simulink model "PIcontroller"  (R2014b)
settings: Solver=ode15s  StartTime=0.0  StopTime=10.0  RelTol=1e-3
settings Model: Creator=c412  LastModifiedBy=c412

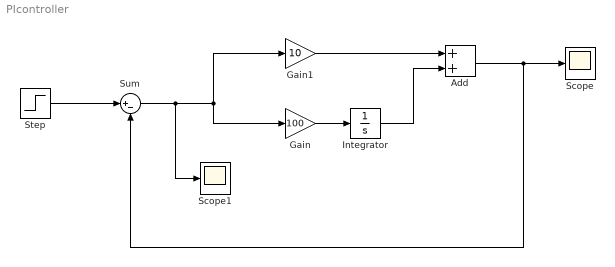
== system PIcontroller ==
  Add : Sum
  Gain : Gain  Gain=100
  Gain1 : Gain  Gain=10
  Integrator : Integrator
  Scope : Scope
  Scope1 : Scope
  Step : Step  SampleTime=0
  Sum : Sum  Inputs=|+-
  wires:
  Gain/1 -> Integrator/1
  Gain1/1 -> Add/1
  Integrator/1 -> Add/2
  Step/1 -> Sum/1
  Add/1 -> Sum/2, Scope/1
  Sum/1 -> Scope1/1, Gain1/1, Gain/1
